simulink model "test_boomCtrl"  (R2015a)
settings: Solver=ode45  StartTime=0.0  StopTime=2  RelTol=1e-3
StartFcn:
  | boomCtrl_param;
values from neighbouring files (symbols this model uses):
  a_boom_yaw_Ctrl = 10*pi/180    (= 0.174532925199)    [boomCtrl_param.m]
  boom_mount_to_center_diagonal = 0.2243    [boomCtrl_param.m]
  l_boom = 1.8161    [boomCtrl_param.m]
undefined symbols (not defined in the file or in its folder): dt_a_dTrunk_boom, dt_fade_boomCtrl, v_dTrunk_boom
libraries: simulink x2
settings Model: Creator=smsong  LastModifiedBy=smsong

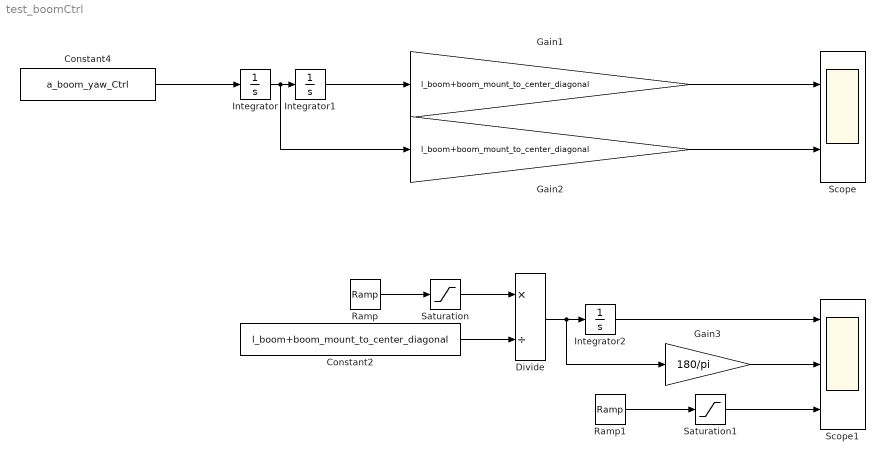
== system test_boomCtrl ==
  Constant2 : Constant  Value=l_boom+boom_mount_to_center_diagonal
  Constant4 : Constant  Value=a_boom_yaw_Ctrl
  Divide : Product  Inputs=*/
  Gain1 : Gain  Gain=l_boom+boom_mount_to_center_diagonal
  Gain2 : Gain  Gain=l_boom+boom_mount_to_center_diagonal
  Gain3 : Gain  Gain=180/pi
  Integrator : Integrator
  Integrator1 : Integrator
  Integrator2 : Integrator
  Ramp : simulink/Sources/Ramp  slope=v_dTrunk_boom/dt_a_dTrunk_boom  start=0  X0=0
  Ramp1 : simulink/Sources/Ramp  slope=-1/dt_fade_boomCtrl  start=dt_a_dTrunk_boom  X0=1
  Saturation : Saturate  UpperLimit=v_dTrunk_boom  LowerLimit=0
  Saturation1 : Saturate  UpperLimit=inf  LowerLimit=0
  Scope : Scope  NumInputPorts=2
      settings: YMin=-5~-5  YMax=5~5
  Scope1 : Scope  NumInputPorts=3
      settings: YMin=-5~-5~-5  YMax=5~5~5
  wires:
  Integrator/1 -> Gain2/1, Integrator1/1
  Integrator1/1 -> Gain1/1
  Constant4/1 -> Integrator/1
  Gain1/1 -> Scope/1
  Gain2/1 -> Scope/2
  Divide/1 -> Gain3/1, Integrator2/1
  Integrator2/1 -> Scope1/1
  Constant2/1 -> Divide/2
  Ramp1/1 -> Saturation1/1
  Ramp/1 -> Saturation/1
  Saturation/1 -> Divide/1
  Saturation1/1 -> Scope1/3
  Gain3/1 -> Scope1/2
